simulink model "model"  (R2023a)
settings: Solver=VariableStepAuto  StartTime=0.0  StopTime=500  RelTol=1e-3
undefined symbols (not defined in the file or in its folder): fs
settings Model: PacingRate=10  Creator=Vram2  LastModifiedBy=Vram2

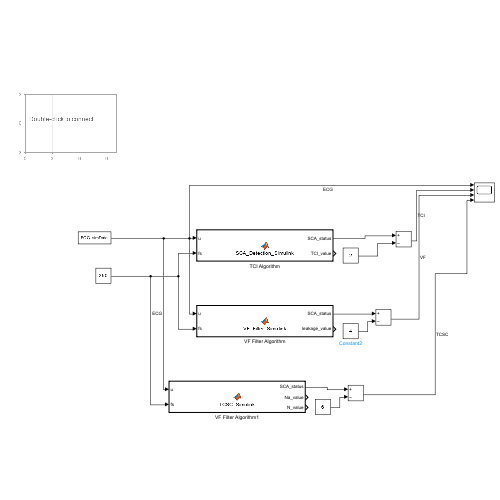
[thumbnail: Simulink's stored preview of the top-level diagram]
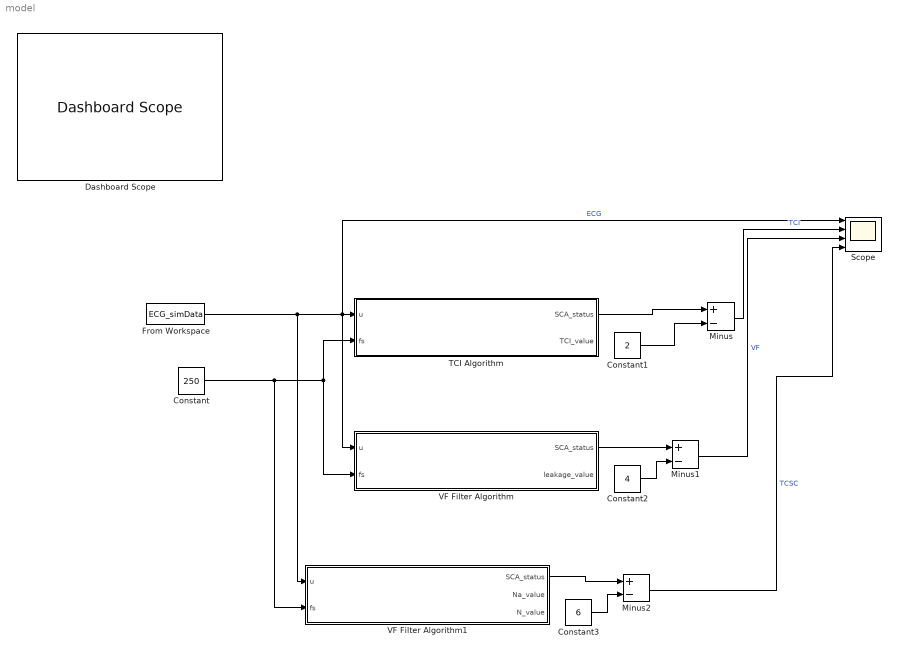
== system model ==
  Constant : Constant  Value=250
  Constant1 : Constant  Value=2
  Constant2 : Constant  Value=4
  Constant3 : Constant  Value=6
  Dashboard Scope : DashboardScope
  From Workspace : FromWorkspace  VariableName=ECG_simData  SampleTime=1/fs
  Minus : Sum  Inputs=+-
  Minus1 : Sum  Inputs=+-
  Minus2 : Sum  Inputs=+-
  Scope : Scope  NumInputPorts=4
  TCI Algorithm : MATLAB Function  TreatAsAtomicUnit=on
  VF Filter Algorithm : MATLAB Function  TreatAsAtomicUnit=on
  VF Filter Algorithm1 : MATLAB Function  TreatAsAtomicUnit=on
  wires:
  TCI Algorithm/1(SCA_status) -> Minus/1
  Minus/1 -> Scope/2  "TCI"
  Constant2/1 -> Minus1/2
  VF Filter Algorithm/1(SCA_status) -> Minus1/1
  Minus1/1 -> Scope/3  "VF"
  Constant1/1 -> Minus/2
  Minus2/1 -> Scope/4  "TCSC"
  VF Filter Algorithm1/1(SCA_status) -> Minus2/1
  Constant/1 -> VF Filter Algorithm1/2(fs), VF Filter Algorithm/2(fs), TCI Algorithm/2(fs)
  Constant3/1 -> Minus2/2
  From Workspace/1 -> VF Filter Algorithm1/1(u), Scope/1, TCI Algorithm/1(u), VF Filter Algorithm/1(u)  "ECG"

== matlab function model/VF Filter Algorithm ==
  data: u input; fs input; SCA_status output; leakage_value output
function [SCA_status, leakage_value] = VF_Filter_Simulink(u, fs)
% VF_Filter_Simulink - Detects VF (Ventricular Fibrillation) from ECG data for use in Simulink
%
% This function is designed to be used in a MATLAB Function block in Simulink
% 
% Inputs:
%   u              - ECG signal value (current sample)
%   fs             - Sampling frequency in Hz
%
% Outputs:
%   SCA_status     - Binary output (1 = SCA detected, 0 = No SCA)
%   leakage_value  - Current leakage value for monitoring
%
% Usage in Simulink:
% 1. Use persistent variables to store signal history
% 2. Analyze accumulated data every second
% 3. Output SCA detection result for Scope block

% Define persistent variables to maintain state between calls
persistent ecg_buffer;       % Buffer to store ECG samples
persistent buffer_index;     % Current index in buffer
persistent last_SCA;         % Last SCA status
persistent last_leakage;     % Last leakage value
persistent buffer_size;      % Size of the buffer (samples per analysis window)
persistent analysis_period;  % How often to run analysis (in samples)
persistent samples_since_analysis; % Counter since last analysis

% Initialize persistent variables on first call
if isempty(ecg_buffer)
    analysis_window_sec = 3;  % Analyze 3 seconds of data
    analysis_period_sec = 1;  % Perform analysis every 1 second
    
    buffer_size = analysis_window_sec * fs;
    analysis_period = analysis_period_sec * fs;
    
    ecg_buffer = zeros(buffer_size, 1);
    buffer_index = 1;
    last_SCA = 0;
    last_leakage = 0.7;  % Default leakage (normal rhythm)
    samples_since_analysis = 0;
end

% Store current ECG sample in buffer (circular buffer)
ecg_buffer(buffer_index) = u;
buffer_index = mod(buffer_index, buffer_size) + 1;
samples_since_analysis = samples_since_analysis + 1;

% Check if it's time to perform analysis (every analysis_period samples)
if samples_since_analysis >= analysis_period && buffer_index > 1
    samples_since_analysis = 0;
    
    % Rearrange buffer to get time-ordered data
    ordered_buffer = [ecg_buffer(buffer_index:end); ecg_buffer(1:buffer_index-1)];
    
    % Run SCA detection algorithm on the buffer
    [SCA_detected, leakage] = OAED_VFfilter_Simulink(ordered_buffer, fs, false);
    
    % Update last detection results
    last_SCA = double(SCA_detected);  % Convert logical to double for Simulink
    last_leakage = leakage;
end

% Output the current SCA status and leakage value
SCA_status = last_SCA;
leakage_value = last_leakage;

end

%% Helper function - Modified version of OAED_VFfilter for Simulink use
function [SCA, l] = OAED_VFfilter_Simulink(ecg, fs, echo)
% Modified version of OAED_VFfilter for use in Simulink
% Input is a single vector of ECG data

if nargin < 3
    echo = false;
end

% Ensure we have enough data for analysis
if length(ecg) < fs
    SCA = false;
    l = 0.7;  % Default value for normal rhythm
    return;
end

% Avoid division by zero and ensure robustness
diff_signal = abs(ecg - [0; ecg(1:end-1)]);
sum_diff = sum(diff_signal);

% Handle edge cases
if sum_diff <= 0 || sum(abs(ecg)) <= 0
    T = fs / 10;  % Default value if calculation fails
    if echo
        disp('Warning: Unable to calculate period, using default');
    end
else
    % Period evaluation
    T = floor(1 + 2*pi * (sum(abs(ecg)) / sum_diff));
    
    % Bound T to reasonable values to prevent extreme results
    T = max(5, min(T, fs));  % Limit between 5 and fs
end

% Leakage evaluation
nt = floor(T/2);

% Ensure we don't exceed array bounds
if nt >= length(ecg)
    nt = floor(length(ecg)/3);  % Use a reasonable default
end

if nt == 0 || length(ecg) <= nt
    l = 0.7;  % Default for normal rhythm
else
    % Calculate leakage properly handling array bounds
    numerator = sum(abs(ecg(nt+1:end) + ecg(1:end-nt)));
    denominator = sum(abs(ecg(nt+1:end)) + abs(ecg(1:end-nt)));
    
    if denominator > 0
        l = numerator / denominator;
    else
        l = 0.7;  % Default for normal rhythm
    end
end

% Rhythm evaluation
l0 = 0.625;
if l > l0
    if echo
        disp('Normal rhythm');
    end
    SCA = false;
else
    if echo
        disp('VF confirmed');
    end
    SCA = true;
end

end

== matlab function model/TCI Algorithm ==
  data: u input; fs input; SCA_status output; TCI_value output
% #codegen

function [SCA_status, TCI_value] = SCA_Detection_Simulink(u, fs)
% SCA_Detection_Simulink - Detects SCA from ECG data for use in Simulink
%
% This function is designed to be used in a MATLAB Function block in Simulink
% 
% Inputs:
%   u          - ECG signal value (current sample)
%   fs         - Sampling frequency in Hz
%
% Outputs:
%   SCA_status - Binary output (1 = SCA detected, 0 = No SCA)
%   TCI_value  - Current TCI value for monitoring
%
% Usage in Simulink:
% 1. Use persistent variables to store signal history
% 2. Analyze accumulated data every second
% 3. Output SCA detection result for Scope block

% Define persistent variables to maintain state between calls
persistent ecg_buffer;       % Buffer to store ECG samples
persistent buffer_index;     % Current index in buffer
persistent last_SCA;         % Last SCA status
persistent last_TCI;         % Last TCI value
persistent buffer_size;      % Size of the buffer (samples per analysis window)
persistent analysis_period;  % How often to run analysis (in samples)
persistent samples_since_analysis; % Counter since last analysis

% Initialize persistent variables on first call
if isempty(ecg_buffer)
    analysis_window_sec = 3;  % Analyze 3 seconds of data
    analysis_period_sec = 1;  % Perform analysis every 1 second
    
    buffer_size = analysis_window_sec * fs;
    analysis_period = analysis_period_sec * fs;
    
    ecg_buffer = zeros(buffer_size, 1);
    buffer_index = 1;
    last_SCA = 0;
    last_TCI = 500;  % Default TCI (normal rhythm)
    samples_since_analysis = 0;
end

% Store current ECG sample in buffer (circular buffer)
ecg_buffer(buffer_index) = u;
buffer_index = mod(buffer_index, buffer_size) + 1;
samples_since_analysis = samples_since_analysis + 1;

% Check if it's time to perform analysis (every analysis_period samples)
if samples_since_analysis >= analysis_period && buffer_index > 1
    samples_since_analysis = 0;
    
    % Rearrange buffer to get time-ordered data
    ordered_buffer = [ecg_buffer(buffer_index:end); ecg_buffer(1:buffer_index-1)];
    
    % Run SCA detection algorithm on the buffer
    [SCA_detected, TCIm, ~] = OAED_TCI_Simulink(ordered_buffer, fs, false);
    
    % Update last detection results
    last_SCA = double(SCA_detected);  % Convert logical to double for Simulink
    last_TCI = TCIm;
end

% Output the current SCA status and TCI value
SCA_status = last_SCA;
TCI_value = last_TCI;

end

%% Helper function - Modified version of OAED_TCI for Simulink use
function [SCA, TCIm, TCI] = OAED_TCI_Simulink(ecg, fs, echo)
% Modified version of OAED_TCI for use in Simulink
% Input is a single vector of ECG data

if nargin < 3
    echo = false;
end

nl = length(ecg);
nsec = 1 * fs;
n = floor(nl/nsec);  % Make sure n is an integer

% If we don't have enough data for a full analysis, return default values
if n < 3
    SCA = false;
    TCIm = 500;
    TCI = [500];
    return;
end

% Find maximum
maxECG = zeros(n,1);
ecg2 = zeros(n,nsec);
for k = 1:n
    ecg2(k,:) = ecg(1 + nsec*(k-1) : nsec*k);
    maxECG(k) = max(abs(ecg2(k,:)));  % Use absolute max for robustness
end

% Binarize the ecg signal
binaryECG = zeros(n,nsec);
for k = 1:n
    if maxECG(k) > 0
        binaryECG(k,:) = (ecg(1 + nsec*(k-1) : nsec*k) > (0.2 * maxECG(k)));
    else
        binaryECG(k,:) = (ecg(1 + nsec*(k-1) : nsec*k) > (1.8 * maxECG(k)));
    end
end

% t evaluation
t = zeros(n,4);
for k = 1:n
    if binaryECG(k,1) == 1
        t(k,2) = 0;
    else
        first_one = find(binaryECG(k,:) == 1, 1, 'first');
        if ~isempty(first_one)
            t(k,2) = (first_one-1) / fs;
        else
            t(k,2) = 0;
        end
    end
    
    if binaryECG(k,end) == 1
        t(k,3) = 0;
    else
        last_one = find(binaryECG(k,:) == 1, 1, 'last');
        if ~isempty(last_one)
            t(k,3) = (nsec - last_one) / fs;
        else
            t(k,3) = 0;
        end
    end
    
    if k == 1
        continue;
    end
    t(k,1) = t(k-1,3);
    t(k-1,4) = t(k,2);
end

% N evaluation
N = zeros(n-2,1);
for k = 2:(n-1)
    for z = 1:nsec-1
        if binaryECG(k,z) ~= binaryECG(k,z+1)
            N(k-1) = N(k-1) + 1;
        end
    end
    N(k-1) = ceil(N(k-1)/2);
    if t(k,2) == 0 && t(k,3) == 0
        N(k-1) = N(k-1) + 1;
    end
end

% TCI evaluation
TCI = zeros(n-2,1);
for k = 2:(n-1)
    if t(k,1) ~= 0
        t12 = t(k,2) / (t(k,1) + t(k,2));
    else
        t12 = 0;
    end
    
    if t(k,3) ~= 0
        t34 = t(k,3) / (t(k,3) + t(k,4));
    else
        t34 = 0;
    end
    
    % Avoid division by zero
    denominator = N(k-1) - 1 + t12 + t34;
    if denominator > 0
        TCI(k-1) = 1000 / denominator;
    else
        TCI(k-1) = 1000;  % Default high value for normal rhythm
    end
end

% Rhythm evaluation
TCIm = mean(TCI);
TCIcrit = 400; % TCI > 400ms => normal sinus rhythm (NSR)

if TCIm <= TCIcrit
    muvf = 105;
    sigmavf = 6.5;
    muvt = 220;
    sigmavt = 16.5;
    alfa = 1 / 100;
    beta = 1 / 100;
    
    F = (1/sigmavf^2) * sum((TCI - muvf).^2) - (1/sigmavt^2) * sum((TCI - muvt).^2);
    FVT = 2*log((1-beta)/alfa) + 2*(n-2)*log(sigmavt/sigmavf);
    FVF = 2*log(beta/(1-alfa)) + 2*(n-2)*log(sigmavt/sigmavf);
    
    if F >= FVT
        if echo
            disp('VT confirmed');
        end
        SCA = true;
    elseif F <= FVF
        if echo
            disp('VF confirmed');
        end
        SCA = true;
    else
        if echo
            disp('Not enough data');
        end
        SCA = false;
    end
else
    if echo
        disp('Normal sinus rhythm');
    end
    SCA = false;
end
end

== matlab function model/VF Filter Algorithm1 ==
  data: u input; fs input; SCA_status output; Na_value output; N_value output
function [SCA_status, Na_value, N_value] = TCSC_Simulink(u, fs)
% TCSC_Simulink - Detects SCA using TCSC algorithm from ECG data for use in Simulink
%
% This function is designed to be used in a MATLAB Function block in Simulink
% 
% Inputs:
%   u         - ECG signal value (current sample)
%   fs        - Sampling frequency in Hz
%
% Outputs:
%   SCA_status - Binary output (1 = SCA detected, 0 = No SCA)
%   Na_value   - Current Na value (average percentage of the signal above threshold)
%   N_value    - Current N value (percentage of the signal above threshold)
%
% Usage in Simulink:
% 1. Use persistent variables to store signal history
% 2. Analyze accumulated data periodically
% 3. Output SCA detection result for Scope block

% Define persistent variables to maintain state between calls
persistent ecg_buffer;           % Buffer to store ECG samples
persistent buffer_index;         % Current index in buffer
persistent last_SCA;             % Last SCA status
persistent last_Na;              % Last Na value
persistent last_N;               % Last N value
persistent buffer_size;          % Size of the buffer (samples)
persistent analysis_period;      % How often to run analysis (in samples)
persistent samples_since_analysis; % Counter since last analysis

% Initialize persistent variables on first call
if isempty(ecg_buffer)
    % TCSC requires at least 3 seconds of data plus additional for analysis window
    analysis_window_sec = 4;     % 4 seconds of data for analysis
    analysis_period_sec = 1;     % Perform analysis every 1 second
    
    buffer_size = analysis_window_sec * fs;
    analysis_period = analysis_period_sec * fs;
    
    ecg_buffer = zeros(buffer_size, 1);
    buffer_index = 1;
    last_SCA = 0;
    last_Na = 0;
    last_N = 0;
    samples_since_analysis = 0;
end

% Store current ECG sample in buffer (circular buffer)
ecg_buffer(buffer_index) = u;
buffer_index = mod(buffer_index, buffer_size) + 1;
samples_since_analysis = samples_since_analysis + 1;

% Check if it's time to perform analysis (every analysis_period samples)
if samples_since_analysis >= analysis_period && buffer_index > 1
    samples_since_analysis = 0;
    
    % Rearrange buffer to get time-ordered data
    ordered_buffer = [ecg_buffer(buffer_index:end); ecg_buffer(1:buffer_index-1)];
    
    % Only run analysis if we have enough data
    if length(ordered_buffer) >= 3 * fs
        % Run SCA detection algorithm on the buffer
        [SCA_detected, Na, N] = OAED_TCSC_Simulink(ordered_buffer, fs, false);
        
        % Update last detection results
        last_SCA = double(SCA_detected);  % Convert logical to double for Simulink
        last_Na = Na;
        last_N = N(end);  % Use the most recent N value for display
    end
end

% Output the current SCA status and Na/N values
SCA_status = last_SCA;
Na_value = last_Na;
N_value = last_N;

end

%% Helper function - Modified version of OAED_TCSC for Simulink use
function [SCA, Na, N] = OAED_TCSC_Simulink(ecg, fs, echo)
% Modified version of OAED_TCSC for use in Simulink
% Input is a single vector of ECG data

if nargin < 3
    echo = false;
end

% Set parameters
Ls = 3;  % Length of analysis window in seconds

% Check if we have enough data
if length(ecg) < Ls * fs
    SCA = false;
    Na = 0;
    N = [0];
    return;
end

% Calculate the length of data in seconds and number of windows
Le = length(ecg)/fs;
ns = Ls * fs;
m = floor(Le - Ls + 1);  % Ensure m is an integer

% Ensure we have at least one complete window
if m < 1
    SCA = false;
    Na = 0;
    N = [0];
    return;
end

% Split signals into windows
ECGsplitted = zeros(m, ns);
for k = 0:m-1
    % Ensure we don't exceed array bounds
    if (k+Ls)*fs <= length(ecg)
        ECGsplitted(1+k, :) = ecg(1 + k*fs : (k+Ls)*fs);
    else
        ECGsplitted(1+k, 1:length(ecg)-k*fs) = ecg(1 + k*fs : end);
    end
end

% Apply cosine window
Lw = 0.25;  % Window length in seconds
nw = floor(Lw*fs);

% Create window functions
W1 = 0.5*(1 - cos(4*pi*(0:1/fs:Lw-1/fs)));
W2 = 0.5*(1 - cos(4*pi*(1/fs+Ls-Lw:1/fs:Ls)));

% Handle edge case where window length calculations result in incompatible sizes
if length(W1) > nw
    W1 = W1(1:nw);
end
if length(W2) > nw
    W2 = W2(1:nw);
end

% Apply windows to ECG segments
ECGfiltered = ECGsplitted;
for k = 1:m
    if nw <= size(ECGfiltered, 2)
        ECGfiltered(k, 1:nw) = ECGsplitted(k, 1:nw) .* W1;
        if nw <= size(ECGfiltered, 2)
            ECGfiltered(k, end-nw+1:end) = ECGsplitted(k, end-nw+1:end) .* W2;
        end
    end
end

% Binarize the ECG signal
binaryECG = zeros(m, ns);
for k = 1:m
    max_val = max(abs(ECGfiltered(k,:)));
    if max_val > 0
        binaryECG(k,:) = (abs(ECGfiltered(k,:)) > 0.2 * max_val);
    end
end

% Calculate N values (percentage of signal above threshold)
N = zeros(m, 1);
for k = 1:m
    N(k) = sum(binaryECG(k,:))/ns * 100;
end

% Calculate average N value
Na = sum(N)/m;

% Rhythm evaluation
Nd = 48;  % Threshold for VF detection (high specificity)
if Na >= Nd
    if echo
        disp('VF confirmed');
    end
    SCA = true;
else
    if echo
        disp('Normal sinus rhythm');
    end
    SCA = false;
end
end
